simulink model "SM_ConvCDCD"  (R2023b)
settings: Solver=ode23s  StartTime=0.0  StopTime=0.01  RelTol=1e-3
values from neighbouring files (symbols this model uses):
  c = 10e-6    (= 1e-05)    [CoCDCD.m]    (also in ConvCDCD.mat)
  d = 0.4    [CoCDCD.m]    (also in ConvCDCD.mat)
  l = 2e-3    (= 0.002)    [CoCDCD.m]    (also in ConvCDCD.mat)
  r = 10    [CoCDCD.m]    (also in ConvCDCD.mat)
  vd = 0.6    [ConvCDCD.mat]

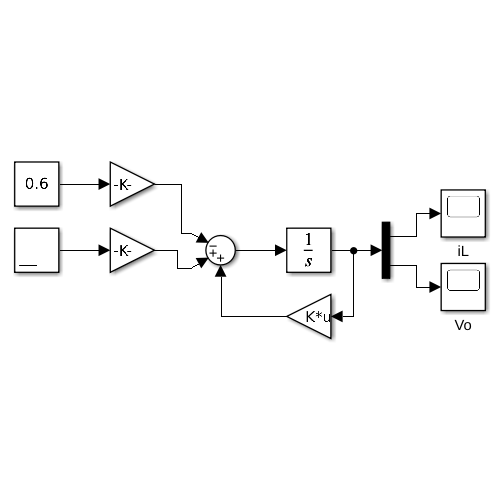
[thumbnail: Simulink's stored preview of the top-level diagram]
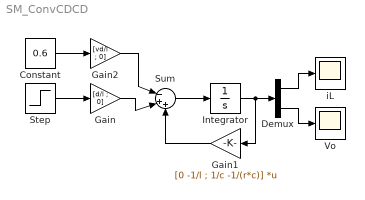
== system SM_ConvCDCD ==
  Constant : Constant  Value=0.6
  Demux : Demux  Outputs=2
  Gain : Gain  Gain=[d/l ; 0]
  Gain1 : Gain  Gain=[0 -1/l ; 1/c -1/(r*c)]  Multiplication=Matrix(K*u)
  Gain2 : Gain  Gain=[vd/l ; 0]
  Integrator : Integrator
  Step : Step  Time=0  After=32  SampleTime=0
  Sum : Sum  Inputs=|-++
  Vo : Scope
  iL : Scope
  wires:
  Sum/1 -> Integrator/1
  Integrator/1 -> Gain1/1, Demux/1
  Demux/2 -> Vo/1
  Demux/1 -> iL/1
  Step/1 -> Gain/1
  Constant/1 -> Gain2/1
  Gain1/1 -> Sum/3
  Gain/1 -> Sum/2
  Gain2/1 -> Sum/1
